simulink model "LED_Toggle"  (R2022b)
settings: Solver=VariableStepAuto  StartTime=0.0  StopTime=10.0  RelTol=1e-3
settings Model: Creator=MAAM  LastModifiedBy=MAAM

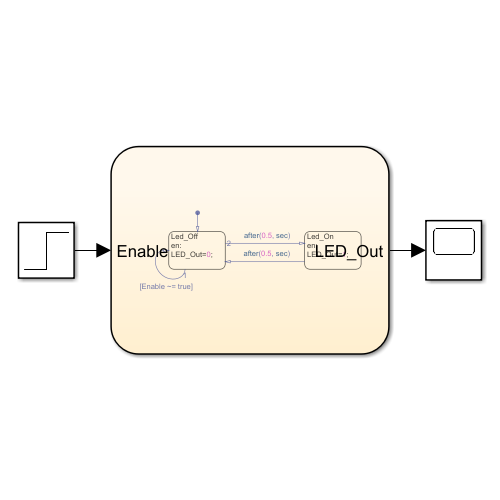
[thumbnail: Simulink's stored preview of the top-level diagram]
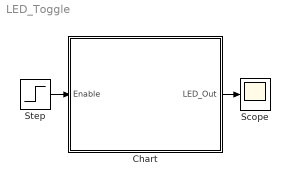
== system LED_Toggle ==
  Chart : Stateflow chart  TreatAsAtomicUnit=on
  Scope : Scope
  Step : Step  Time=5  OutDataTypeStr=single  SampleTime=0
  wires:
  Step/1 -> Chart/1(Enable)
  Chart/1(LED_Out) -> Scope/1

== stateflow chart LED_Toggle/Chart ==
  state Led_Off
    en:
    LED_Out=0;
  state Led_On
    en:
    LED_Out=1;
  (default) -> Led_Off
  Led_Off -> Led_On [order 2] : after(0.5, sec)
  Led_Off -> Led_Off [order 1] : [Enable ~= true]
  Led_On -> Led_Off : after(0.5, sec)
  data: Enable input; LED_Out output
